simulink model "Competition"  (Simulink 7.0)
settings: Solver=ode23tb  StartTime=0.0  StopTime=10000.0  MaxStep=1  RelTol=1e-3
undefined symbols (not defined in the file): DiscIntNeverNeededParam
libraries: LemmingToolbox x4, simulink x2
settings Model: Creator=langmo  LastModifiedBy=langmo

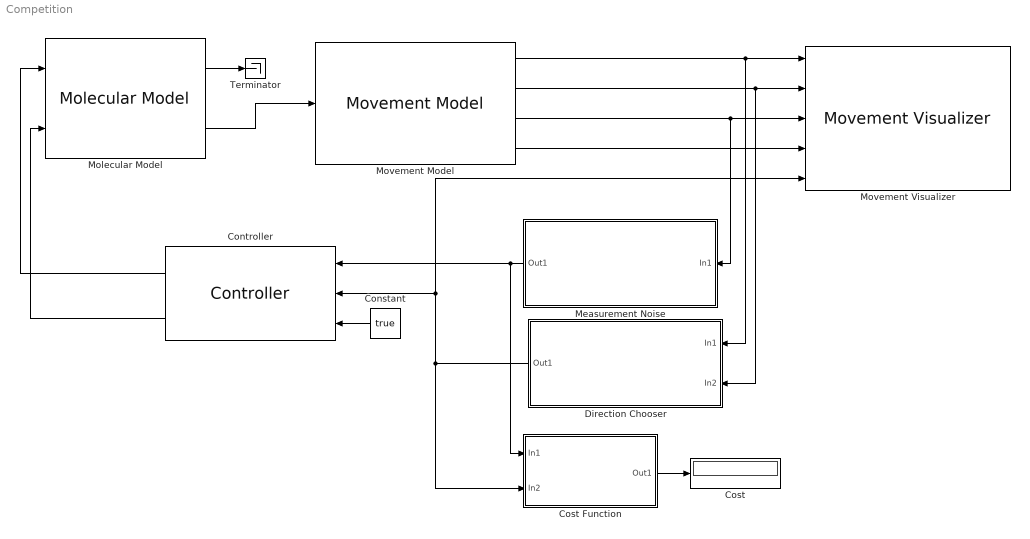
== system Competition ==
  Constant : Constant  Orientation=left  Value=true  OutDataType=sfix(16)  OutScaling=2^0
  Controller : LemmingToolbox/Controller  Orientation=left  sampleTimes=[0.3, 0]  controller=@controllerHysteresis
  Cost : Display
  Cost Function : Subsystem
      mask Display:
      | text(0.3,0.1,'Cost Function');
      | color('blue');
      | port_label('input', 1, 'phi_is');
      | port_label('input', 2, 'phi_sh');
      | color('red');
      | port_label('output', 1, 'Performance');
  Direction Chooser : Subsystem  Orientation=left
      mask Display:
      | text(0.3,0.1,'Direction Chooser');
      | color('blue');
      | port_label('input', 1, 'X-Pos');
      | port_label('input', 2, 'Y-Pos');
      | port_label('output', 1, 'phi_sh');
  Measurement Noise : Subsystem  Orientation=left
      mask Display:
      | text(0.3,0.1,'Measurement Noise');
      | color('blue');
      | port_label('input', 1, 'phi_is');
      | port_label('output', 1, 'phi_is');
  Molecular Model : LemmingToolbox/Molecular Model  molecModel=Spiro  controlledCheSpecies=CheY  cheSpeciesAttachedTo=CheX-PIF3 & PhyB-Anker  asp=1e-3  useOrgParameters=off  CheX=42  AnkerProt=57  Anker=80
  Movement Model : LemmingToolbox/Movement Model  imageDim=[1344,1024]  binning=2  pixelSize=6.45 / 40  initialCondition=[0, 0, 0]  sampleTimes=[0.03, 0]
  Movement Visualizer : LemmingToolbox/Movement Visualizer  numPoints=1000  sampleTimes=[0.3, 0.1]
  Terminator : Terminator
  wires:
  Molecular Model/2 -> Movement Model/1
  Molecular Model/1 -> Terminator/1
  Movement Model/3 -> Measurement Noise/1(In1), Movement Visualizer/3
  Cost Function/1(Out1) -> Cost/1
  Constant/1 -> Controller/3
  Measurement Noise/1(Out1) -> Controller/1, Cost Function/1(In1)
  Movement Model/1 -> Direction Chooser/1(In1), Movement Visualizer/1
  Movement Model/2 -> Direction Chooser/2(In2), Movement Visualizer/2
  Movement Model/4 -> Movement Visualizer/4
  Direction Chooser/1(Out1) -> Controller/2, Movement Visualizer/5, Cost Function/2(In2)
  Controller/1 -> Molecular Model/1
  Controller/2 -> Molecular Model/2

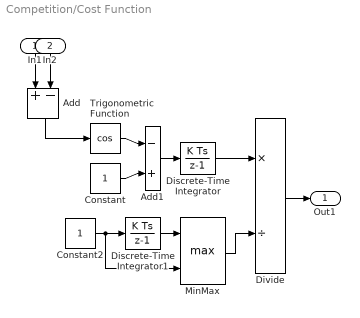
== system Competition/Cost Function ==
  In1 : Inport  Orientation=down
  In2 : Inport  Orientation=down  Port=2
  Add : Sum  Orientation=down  Inputs=+-  OutDataType=sfix(16)  OutScaling=2^-10
  Add1 : Sum  Inputs=-|+  OutDataType=sfix(16)  OutScaling=2^-10
  Constant : Constant  OutDataType=sfix(16)  OutScaling=2^0
  Constant2 : Constant  OutDataType=sfix(16)  OutScaling=2^0  SampleTime=[0.3,0]
  Discrete-Time Integrator : DiscreteIntegrator  SampleTime=0.3  OutDataType=sfix(16)  OutScaling=2^0  ICPrevOutput=DiscIntNeverNeededParam  ICPrevScaledInput=DiscIntNeverNeededParam
  Discrete-Time Integrator1 : DiscreteIntegrator  SampleTime=-1  OutDataType=sfix(16)  OutScaling=2^0  ICPrevOutput=DiscIntNeverNeededParam  ICPrevScaledInput=DiscIntNeverNeededParam
  Divide : Product  Inputs=*/  OutDataType=sfix(16)  OutScaling=2^-10
  MinMax : MinMax  Function=max  Inputs=2  OutDataType=sfix(16)  OutScaling=2^0
  Trigonometric Function : Trigonometry  Operator=cos
  Out1 : Outport
  wires:
  Add/1 -> Trigonometric Function/1
  Trigonometric Function/1 -> Add1/1
  Constant/1 -> Add1/2
  Add1/1 -> Discrete-Time Integrator/1
  Constant2/1 -> Discrete-Time Integrator1/1, MinMax/2
  Discrete-Time Integrator/1 -> Divide/1
  In1/1 -> Add/1
  In2/1 -> Add/2
  Divide/1 -> Out1/1
  MinMax/1 -> Divide/2
  Discrete-Time Integrator1/1 -> MinMax/1

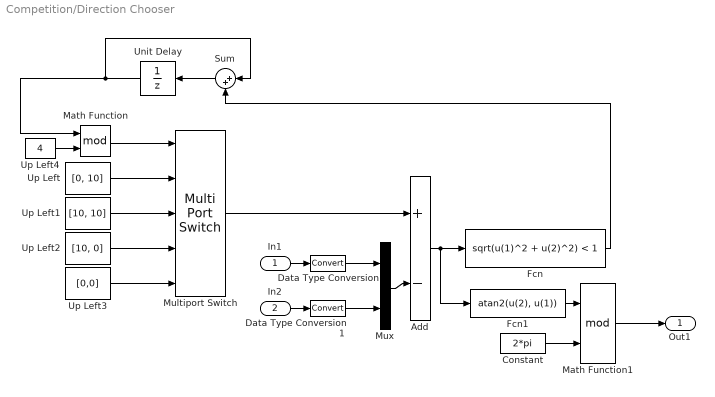
== system Competition/Direction Chooser ==
  In1 : Inport
  In2 : Inport  Port=2
  Add : Sum  Inputs=+-  OutDataType=sfix(16)  OutScaling=2^-10
  Constant : Constant  Value=2*pi  OutDataType=sfix(16)  OutScaling=2^0
  Data Type Conversion : DataTypeConversion  OutDataTypeMode=double  OutDataType=sfix(16)  OutScaling=2^0  SampleTime=0.3
  Data Type Conversion1 : DataTypeConversion  OutDataTypeMode=double  OutDataType=sfix(16)  OutScaling=2^0  SampleTime=0.3
  Fcn : Fcn  Expr=sqrt(u(1)^2 + u(2)^2) < 1
  Fcn1 : Fcn  Expr=atan2(u(2), u(1))
  Math Function : Math  Operator=mod  OutDataType=sfix(16)  OutScaling=2^0  SaturateOnIntegerOverflow=on
  Math Function1 : Math  Operator=mod  OutDataType=sfix(16)  OutScaling=2^0  SaturateOnIntegerOverflow=on
  Multiport Switch : MultiPortSwitch  zeroidx=on  OutDataType=sfix(16)  OutScaling=2^0
  Mux : Mux  Inputs=2
  Sum : Sum  Orientation=left  Inputs=|++  OutDataType=sfix(16)  OutScaling=2^0
  Unit Delay : UnitDelay  Orientation=left  SampleTime=0.3
  Up Left : Constant  Value=[0, 10]  OutDataType=sfix(16)  OutScaling=2^0
  Up Left1 : Constant  Value=[10, 10]  OutDataType=sfix(16)  OutScaling=2^0
  Up Left2 : Constant  Value=[10, 0]  OutDataType=sfix(16)  OutScaling=2^0
  Up Left3 : Constant  Value=[0,0]  OutDataType=sfix(16)  OutScaling=2^0
  Up Left4 : Constant  Value=4  OutDataType=sfix(16)  OutScaling=2^0
  Out1 : Outport
  wires:
  Up Left/1 -> Multiport Switch/2
  Up Left3/1 -> Multiport Switch/5
  Up Left2/1 -> Multiport Switch/4
  Up Left1/1 -> Multiport Switch/3
  In2/1 -> Data Type Conversion1/1
  In1/1 -> Data Type Conversion/1
  Sum/1 -> Unit Delay/1
  Unit Delay/1 -> Sum/1, Math Function/1
  Up Left4/1 -> Math Function/2
  Math Function/1 -> Multiport Switch/1
  Multiport Switch/1 -> Add/1
  Mux/1 -> Add/2
  Add/1 -> Fcn/1, Fcn1/1
  Fcn/1 -> Sum/2
  Data Type Conversion/1 -> Mux/1
  Data Type Conversion1/1 -> Mux/2
  Fcn1/1 -> Math Function1/1
  Constant/1 -> Math Function1/2
  Math Function1/1 -> Out1/1

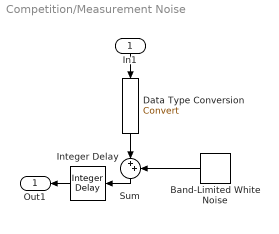
== system Competition/Measurement Noise ==
  In1 : Inport  Orientation=down
  Band-Limited White Noise : simulink/Sources/Band-Limited White Noise  Orientation=left  SystemSampleTime=-1  Cov=[0.004]  Ts=0.3  seed=[23341]
  Data Type Conversion : DataTypeConversion  Orientation=down  OutDataTypeMode=double  OutDataType=sfix(16)  OutScaling=2^0  SampleTime=0.3
  Integer Delay : simulink/Discrete/Integer Delay  Orientation=left  vinit=0.0  samptime=-1  NumDelays=3
  Sum : Sum  Orientation=down  Inputs=|++  OutDataType=sfix(16)  OutScaling=2^0
  Out1 : Outport  Orientation=left
  wires:
  Band-Limited White Noise/1 -> Sum/2
  Data Type Conversion/1 -> Sum/1
  Sum/1 -> Integer Delay/1
  In1/1 -> Data Type Conversion/1
  Integer Delay/1 -> Out1/1
